simulink model "computeFnull"  (Simulink 7.7)
settings: Solver=FixedStepDiscrete  StartTime=0.0  StopTime=2  FixedStep=0.01  RelTol=1e-3
PreLoadFcn:
  | robotName = 'icubGazeboSim';
  | localName = 'SimulinkiCubGazeboSim';
InitFcn:
  | robotName = 'icubGazeboSim';
  | localName = 'SimulinkiCubGazeboSim';
libraries: WBCLibrary x16
settings Model: Creator=iron  LastModifiedBy=iron

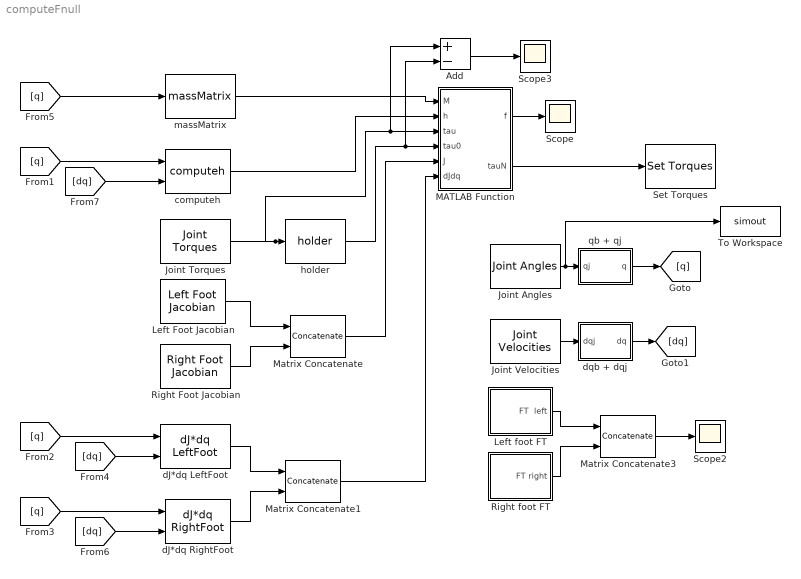
== system computeFnull ==
  Add : Sum  Inputs=+-
  Joint Angles : WBCLibrary/wholeBodyStates/Joint Angles  SystemSampleTime=-1  robotName=robotName  localName=localName
  Joint Torques : WBCLibrary/wholeBodyStates/Joint Torques  SystemSampleTime=-1  robotName=robotName  localName=localName
  Joint Velocities : WBCLibrary/wholeBodyStates/Joint Velocities  SystemSampleTime=-1  robotName=robotName  localName=localName
  Left Foot Jacobian : WBCLibrary/wholeBodyModel/Jacobians/Left Foot Jacobian  SystemSampleTime=-1  robotName=robotName  localName=localName
  Left foot FT : Subsystem
  MATLAB Function : Stateflow chart  TreatAsAtomicUnit=on
  Matrix Concatenate : Concatenate  Mode=Multidimensional array
  Matrix Concatenate1 : Concatenate  Mode=Multidimensional array
  Matrix Concatenate3 : Concatenate  Mode=Multidimensional array
  Right Foot Jacobian : WBCLibrary/wholeBodyModel/Jacobians/Right Foot Jacobian  SystemSampleTime=-1  robotName=robotName  localName=localName
  Right foot FT : Subsystem
  Scope : Scope
      settings: TimeRange=0.9  YMin=-20  YMax=160
  Scope2 : Scope
      settings: TimeRange=0.9  YMin=-10  YMax=120
  Scope3 : Scope
      settings: TimeRange=0.9  YMin=-0.025  YMax=0.225  SaveName=ScopeData3
  Set Torques : WBCLibrary/wholeBodyActuators/Set Torques  SystemSampleTime=-1  val=6  robotName=robotName  localName=localName
  To Workspace : ToWorkspace  VariableName=simout  SampleTime=-1  SaveFormat=Structure
  computeh : WBCLibrary/wholeBodyModel/Dynamics/computeh  SystemSampleTime=-1  val=7  robotname=robotName  localname=localName
  dJ*dq LeftFoot : WBCLibrary/wholeBodyModel/Dynamics/dJ*dq LeftFoot  SystemSampleTime=-1  val=9  robotName=robotName  localName=localName
  dJ*dq RightFoot : WBCLibrary/wholeBodyModel/Dynamics/dJ*dq RightFoot  SystemSampleTime=-1  val=9  robotName=robotName  localName=localName
  dqb + dqj : Subsystem
  holder : WBCLibrary/Utilities/holder  SystemSampleTime=-1
  massMatrix : WBCLibrary/wholeBodyModel/Dynamics/massMatrix  SystemSampleTime=-1  val=8  robotname=robotName  localname=localName
  qb + qj : Subsystem
  wires:
  massMatrix/1 -> MATLAB Function/1(M)
  computeh/1 -> MATLAB Function/2(h)
  Left Foot Jacobian/1 -> Matrix Concatenate/1
  Right Foot Jacobian/1 -> Matrix Concatenate/2
  Matrix Concatenate/1 -> MATLAB Function/5(J)
  dJ*dq LeftFoot/1 -> Matrix Concatenate1/1
  dJ*dq RightFoot/1 -> Matrix Concatenate1/2
  Matrix Concatenate1/1 -> MATLAB Function/6(dJdq)
  MATLAB Function/1(f) -> Scope/1
  Left foot FT/1(FT  left) -> Matrix Concatenate3/1
  Right foot FT/1(FT right) -> Matrix Concatenate3/2
  Matrix Concatenate3/1 -> Scope2/1
  Joint Angles/1 -> qb + qj/1(qj), To Workspace/1
  Joint Velocities/1 -> dqb + dqj/1(dqj)
  qb + qj/1(q) -> [q]
  dqb + dqj/1(dq) -> [dq]
  [q] -> massMatrix/1
  [q] -> computeh/1
  [q] -> dJ*dq LeftFoot/1
  [q] -> dJ*dq RightFoot/1
  [dq] -> computeh/2
  [dq] -> dJ*dq LeftFoot/2
  [dq] -> dJ*dq RightFoot/2
  MATLAB Function/2(tauN) -> Set Torques/1
  holder/1 -> MATLAB Function/4(tau0), Add/2
  Joint Torques/1 -> holder/1, MATLAB Function/3(tau), Add/1
  Add/1 -> Scope3/1

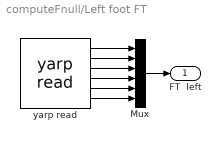
== system computeFnull/Left foot FT ==
  Mux : Mux  Inputs=6
  yarp read : WBCLibrary/Utilities/yarp read  from=['/' robotName '/left_foot/analog:o']  to='/left_foot/FT'  num=6
  FT  left : Outport
  wires:
  yarp read/1 -> Mux/1
  yarp read/2 -> Mux/2
  yarp read/3 -> Mux/3
  yarp read/4 -> Mux/4
  yarp read/5 -> Mux/5
  yarp read/6 -> Mux/6
  Mux/1 -> FT  left/1

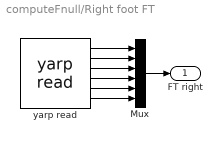
== system computeFnull/Right foot FT ==
  Mux : Mux  Inputs=6
  yarp read : WBCLibrary/Utilities/yarp read  from=['/' robotName '/right_foot/analog:o']  to='/right_foot/FT'  num=6
  FT right : Outport
  wires:
  yarp read/1 -> Mux/1
  yarp read/2 -> Mux/2
  yarp read/3 -> Mux/3
  yarp read/4 -> Mux/4
  yarp read/5 -> Mux/5
  yarp read/6 -> Mux/6
  Mux/1 -> FT right/1

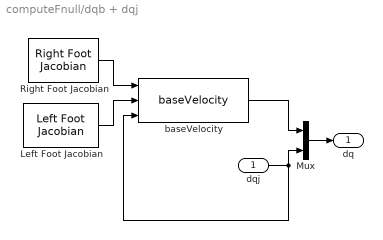
== system computeFnull/dqb + dqj ==
  dqj : Inport
  Left Foot Jacobian : WBCLibrary/wholeBodyModel/Jacobians/Left Foot Jacobian  SystemSampleTime=-1  robotName=robotName  localName=localName
  Mux : Mux  Inputs=2
  Right Foot Jacobian : WBCLibrary/wholeBodyModel/Jacobians/Right Foot Jacobian  SystemSampleTime=-1  robotName=robotName  localName=localName
  baseVelocity : WBCLibrary/Utilities/baseVelocity  SystemSampleTime=-1
  dq : Outport
  wires:
  Left Foot Jacobian/1 -> baseVelocity/2
  Right Foot Jacobian/1 -> baseVelocity/1
  baseVelocity/1 -> Mux/1
  dqj/1 -> baseVelocity/3, Mux/2
  Mux/1 -> dq/1

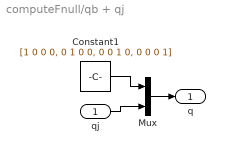
== system computeFnull/qb + qj ==
  qj : Inport
  Constant1 : Constant  Value=[1 0 0 0, 0 1 0 0, 0 0 1 0, 0 0 0 1]
  Mux : Mux  Inputs=2
  q : Outport
  wires:
  Mux/1 -> q/1
  qj/1 -> Mux/2
  Constant1/1 -> Mux/1

== matlab function MATLAB Function ==
  data: M input double; f output double; h input double; tau input double; tau0 input double; J input double; dJdq input double; tauN output double
function [f, tauN] = fcn(M, h, tau, tau0, J, dJdq)

% Francesco Nori
% Genova 6 Marzo 2014
% CODYCO project
%
% This code computes the forces f acting on a kinematic chain
% subject to a set of constraints. The kinematic chain dynamics
% are described as follows:
%
% M d2q + h - J' f = tau  
%
% The constraints are described in a differential form:
%
% J dq = 0
%
% whose derivative is:
%
% dJ dq  + J d2q = 0
%
% The output tauN belongs to the null space of f. The projector
% on the null space of f is computed in different forms. First
% it is observed that:
% 
% f = -(J*Minv*J')^(-1)(J*Minv*(S'*tau - h)+ dJdq); 
%
% and therefore given that f = A*tau + b, the nullspace for f
% can be constructed as (I - pinv(A)*A). Moreover since we have
% f = (J*Minv*J')^(-1)*B*tau + b we can also compute vectors in
% the nullspace of f with (I - pinv(B)*B). Finally, as reported
% in Del Prete, Ph.D. thesis we can also express the very same
% matrix as Nj_inv*(eye(25) - pinv(C) * C).

Minv = inv(M);

Mb     = M(1:6 ,  1:6);
Mj     = M(7:31, 7:31);
Mbj    = M(1:6 , 7:31);
Nj_inv = Mj - Mbj' * Mb^(-1) * Mbj;
Nj     = Minv(7:31, 7:31);

Sbar = [-Mb^(-1) * Mbj; eye(25)];
S    = [zeros(25,6) eye(25)];

f = -(J*Minv*J')\(J*Minv*(S'*tau - h)+ dJdq); 

% A = (J*Minv*J')\(J*Minv*S');
% tauN = tau0 + (eye(25) - pinv(A)*A)*(ones(size(tau)).*10);

% V  = Nj_inv*Nj_inv;
% B  = J*Minv*S';
% Bp = V*B'/(B*V*B'); 
% tauN = tau0 + (eye(25) - Bp*B)*(ones(size(tau)));

C = J*Sbar;
tauN = tau0 + Nj_inv*(eye(25) - pinv(C) * C)*Nj*(ones(size(tau)));
% norm(Nj_inv*(eye(25) - pinv(C) * C)*Nj - (eye(25) - Bp*B));
% tauN = zeros(size(tauN));
